simulink model "AeroPistonEngineSimulator"  (R2026a)
settings: Solver=VariableStepAuto  StopTime=100.0
model workspace (MAT data in the model file):
  linear_friction_constant = 0.001
undefined symbols (not defined in the file or in its folder): C_oil, CHT_capacity, EGT_tau, Fault_ID, friction_a, friction_b, J_engine, k_c, k_h, k_oil_cool, k_oil_heat, k_oil_pressure_rpm, k_oil_pressure_temp, RPM_max, T_max
libraries: simulink x17
settings Model: Creator=ambar  LastModifiedBy=skm
settings DataIOCC: LoadExternalInput=on

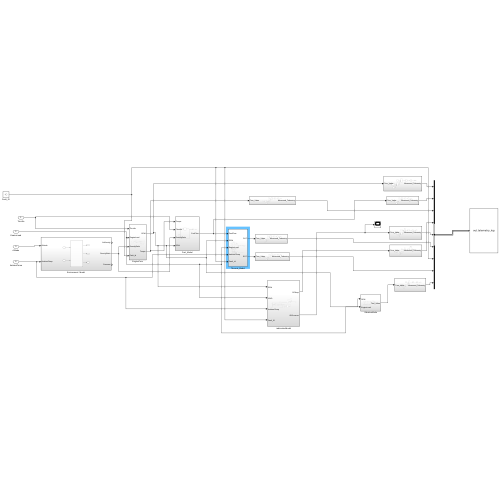
[thumbnail: Simulink's stored preview of the top-level diagram]
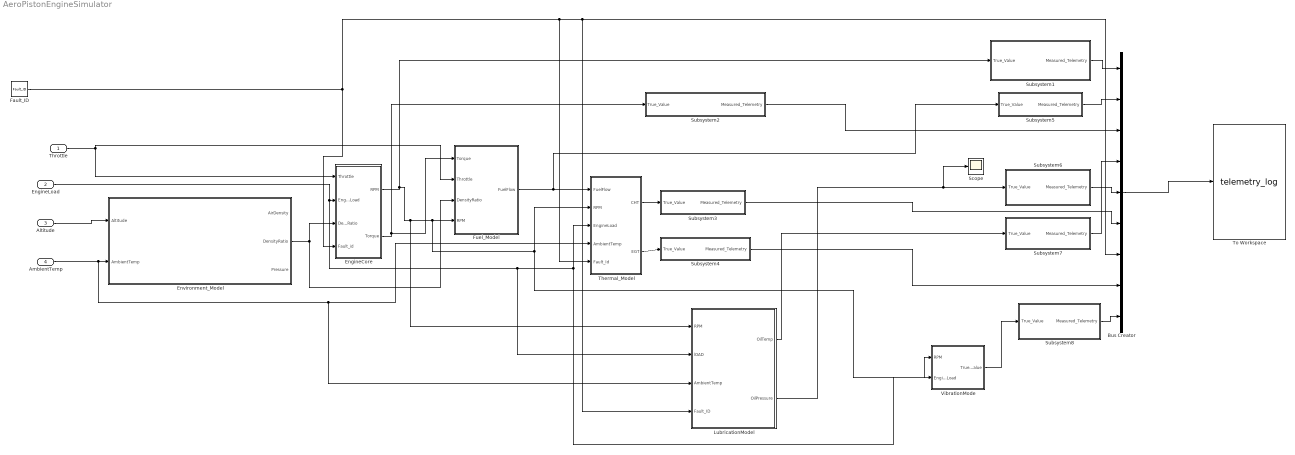
== system AeroPistonEngineSimulator ==
  Throttle : Inport
  EngineLoad : Inport  Port=2
  Altitude : Inport  Port=3
  AmbientTemp : Inport  Port=4
  Bus Creator : BusCreator  Inputs=9
  EngineCore : Subsystem
  Environment_Model : Subsystem
  Fault_ID : Constant  Value=Fault_ID
  Fuel_Model : Subsystem
  LubricationModel : Subsystem
  Scope : Scope
      settings: ActiveDisplayYMinimum=-7.3974032772630345  ActiveDisplayYMaximum=74.925308630368761  DataLoggingVariableName=ScopeData4
  Subsystem1 : Subsystem
  Subsystem2 : Subsystem
  Subsystem3 : Subsystem
  Subsystem4 : Subsystem
  Subsystem5 : Subsystem
  Subsystem6 : Subsystem
  Subsystem7 : Subsystem
  Subsystem8 : Subsystem
  Thermal_Model : Subsystem
  To Workspace : ToWorkspace  VariableName=telemetry_log  SaveFormat=Timeseries  SampleTime=-1
  VibrationMode : Subsystem
  wires:
  Altitude/1 -> Environment_Model/1(Altitude)
  AmbientTemp/1 -> LubricationModel/3(AmbientTemp), Thermal_Model/4(AmbientTemp), Environment_Model/2(AmbientTemp)
  Environment_Model/2(DensityRatio) -> Fuel_Model/3(DensityRatio), EngineCore/3(DensityRatio)
  EngineCore/1(RPM) -> Subsystem1/1(True_Value), LubricationModel/1(RPM), VibrationMode/1(RPM), Thermal_Model/2(RPM), Fuel_Model/4(RPM)
  EngineCore/2(Torque) -> Subsystem2/1(True_Value), Fuel_Model/1(Torque)
  Fuel_Model/1(FuelFlow) -> Subsystem5/1(True_Value), Thermal_Model/1(FuelFlow)
  Throttle/1 -> Fuel_Model/2(Throttle), EngineCore/1(Throttle)
  EngineLoad/1 -> LubricationModel/2(lOAD), Thermal_Model/3(EngineLoad), VibrationMode/2(EngineLoad), EngineCore/2(EngineLoad)
  Thermal_Model/1(CHT) -> Subsystem3/1(True_Value)
  Thermal_Model/2(EGT) -> Subsystem4/1(True_Value)
  LubricationModel/1(OilTemp) -> Subsystem7/1(True_Value)
  VibrationMode/1(True_Value) -> Subsystem8/1(True_Value)
  Subsystem8/1(Measured_Telemetry) -> Bus Creator/9
  Subsystem6/1(Measured_Telemetry) -> Bus Creator/5
  Subsystem7/1(Measured_Telemetry) -> Bus Creator/4
  Subsystem5/1(Measured_Telemetry) -> Bus Creator/2
  Subsystem1/1(Measured_Telemetry) -> Bus Creator/1
  Subsystem4/1(Measured_Telemetry) -> Bus Creator/8
  Subsystem3/1(Measured_Telemetry) -> Bus Creator/6
  Bus Creator/1 -> To Workspace/1
  Subsystem2/1(Measured_Telemetry) -> Bus Creator/3
  Fault_ID/1 -> Thermal_Model/5(Fault_Id), Bus Creator/7, LubricationModel/4(Fault_ID), EngineCore/4(Fault_id)
  LubricationModel/2(OilPressure) -> Scope/1, Subsystem6/1(True_Value)

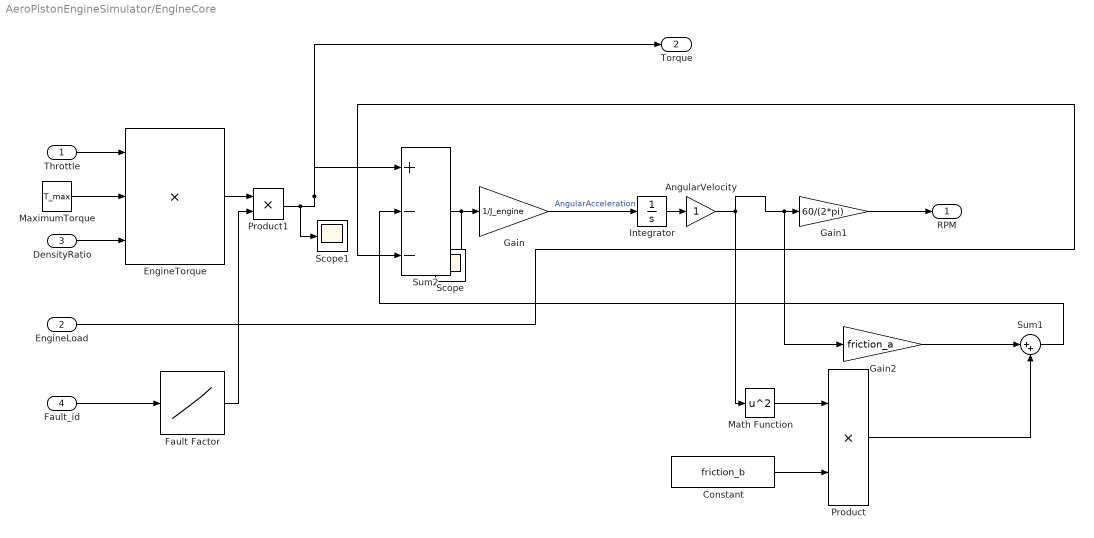
== system AeroPistonEngineSimulator/EngineCore ==
  Throttle : Inport
  EngineLoad : Inport  Port=2
  DensityRatio : Inport  Port=3
  Fault_id : Inport  Port=4
  AngularVelocity : Gain
  Constant : Constant  Value=friction_b
  EngineTorque : Product  Inputs=3
  Fault Factor : Lookup_n-D  NumberOfTableDimensions=1  BreakpointsForDimension1=[0 1 2 3 4]  Table=[1 0.65 1 1 1]  InternalRulePriority=Speed  RndMeth=Simplest
  Gain : Gain  Gain=1/J_engine
  Gain1 : Gain  Gain=60/(2*pi)
  Gain2 : Gain  Gain=friction_a
  Integrator : Integrator
  Math Function : Math  Operator=square
  MaximumTorque : Constant  Value=T_max  VectorParams1D=off
  Product : Product
  Product1 : Product
  Scope : Scope
      settings: ActiveDisplayYMinimum=-1.14558689108388  ActiveDisplayYMaximum=10.310282019757746  DataLoggingVariableName=ScopeData5
  Scope1 : Scope
      settings: ActiveDisplayYMinimum=-1  ActiveDisplayYMaximum=1  DataLoggingVariableName=ScopeData6
  Sum1 : Sum  Inputs=|++
  Sum2 : Sum  Inputs=|+--
  RPM : Outport
  Torque : Outport  Port=2
  wires:
  Throttle/1 -> EngineTorque/1
  DensityRatio/1 -> EngineTorque/3
  MaximumTorque/1 -> EngineTorque/2
  EngineTorque/1 -> Product1/1
  EngineLoad/1 -> Sum2/3
  Sum2/1 -> Scope/1, Gain/1
  Gain/1 -> Integrator/1  "AngularAcceleration"
  Gain1/1 -> RPM/1
  Integrator/1 -> AngularVelocity/1
  AngularVelocity/1 -> Gain1/1, Gain2/1, Math Function/1
  Math Function/1 -> Product/1
  Constant/1 -> Product/2
  Gain2/1 -> Sum1/1
  Product/1 -> Sum1/2
  Sum1/1 -> Sum2/2
  Fault_id/1 -> Fault Factor/1
  Product1/1 -> Scope1/1, Torque/1, Sum2/1
  Fault Factor/1 -> Product1/2

== system AeroPistonEngineSimulator/Environment_Model ==
  Altitude : Inport
  AmbientTemp : Inport  Port=2
  MATLAB Function : MATLAB Function  TreatAsAtomicUnit=on
  AirDensity : Outport
  DensityRatio : Outport  Port=2
  Pressure : Outport  Port=3
  wires:
  Altitude/1 -> MATLAB Function/1(altitude)
  AmbientTemp/1 -> MATLAB Function/2(temp_celsius)
  MATLAB Function/2(density) -> AirDensity/1
  MATLAB Function/3(density_ratio) -> DensityRatio/1
  MATLAB Function/1(pressure) -> Pressure/1

== system AeroPistonEngineSimulator/Fuel_Model ==
  Torque : Inport
  Throttle : Inport  Port=2
  DensityRatio : Inport  Port=3
  RPM : Inport  Port=4
  2-D Lookup Table : Lookup_n-D  BreakpointsForDimension1=[1500, 3000, 5000, 7000]  BreakpointsForDimension2=[0.2, 0.5, 0.8, 1.0]  Table=[0.5 0.8 1.2 1.5; 1.0 1.5 2.0 2.5; 1.8 2.2 2.8 3.5; 2.5 3.0 3.8 4.5]  InternalRulePriority=Speed  RndMeth=Simplest
      settings: InputPortMap=u0,u1
  Product : Product
  FuelFlow : Outport
  wires:
  RPM/1 -> 2-D Lookup Table/1
  Throttle/1 -> 2-D Lookup Table/2
  2-D Lookup Table/1 -> Product/1
  DensityRatio/1 -> Product/2
  Product/1 -> FuelFlow/1

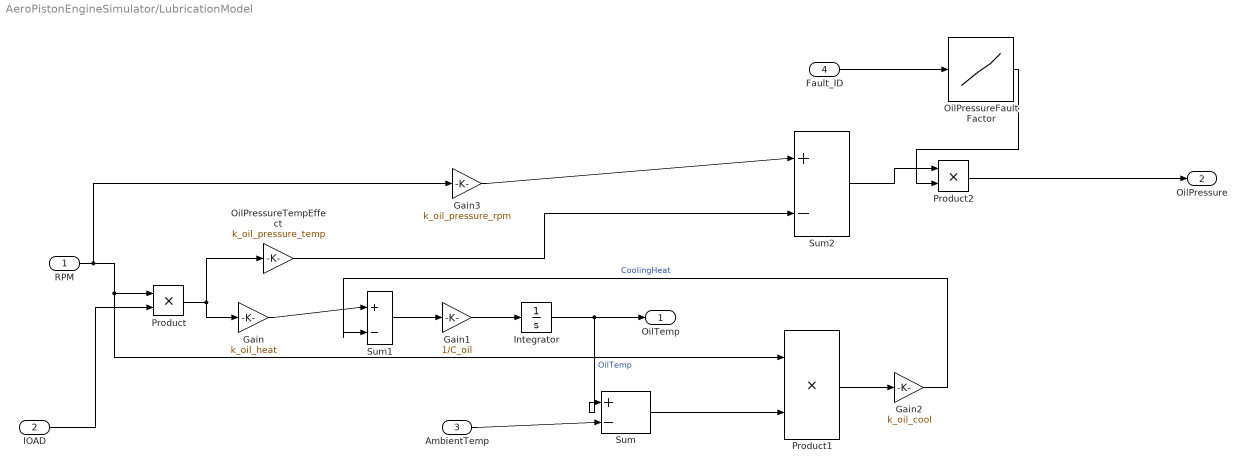
== system AeroPistonEngineSimulator/LubricationModel ==
  RPM : Inport
  lOAD : Inport  Port=2
  AmbientTemp : Inport  Port=3
  Fault_ID : Inport  Port=4
  Gain : Gain  Gain=k_oil_heat
  Gain1 : Gain  Gain=1/C_oil
  Gain2 : Gain  Gain=k_oil_cool
  Gain3 : Gain  Gain=k_oil_pressure_rpm
  Integrator : Integrator  InitialCondition=25
  OilPressureFault Factor : Lookup_n-D  NumberOfTableDimensions=1  BreakpointsForDimension1=[0 1 2 3 4]  Table=[1 1 1 0.2 1]  InternalRulePriority=Speed  RndMeth=Simplest
  OilPressureTempEffect : Gain  Gain=k_oil_pressure_temp
  Product : Product
  Product1 : Product
  Product2 : Product
  Sum : Sum  Inputs=|+-
  Sum1 : Sum  Inputs=|+-
  Sum2 : Sum  Inputs=|+-
  OilTemp : Outport
  OilPressure : Outport  Port=2
  wires:
  RPM/1 -> Gain3/1, Product1/1, Product/1
  lOAD/1 -> Product/2
  Product/1 -> OilPressureTempEffect/1, Gain/1
  AmbientTemp/1 -> Sum/2
  Gain/1 -> Sum1/1
  Sum1/1 -> Gain1/1
  Gain1/1 -> Integrator/1
  Integrator/1 -> Sum/1, OilTemp/1  "OilTemp"
  Sum/1 -> Product1/2
  Product1/1 -> Gain2/1
  Gain2/1 -> Sum1/2  "CoolingHeat"
  Gain3/1 -> Sum2/1
  Product2/1 -> OilPressure/1
  OilPressureTempEffect/1 -> Sum2/2
  Sum2/1 -> Product2/1
  Fault_ID/1 -> OilPressureFault Factor/1
  OilPressureFault Factor/1 -> Product2/2

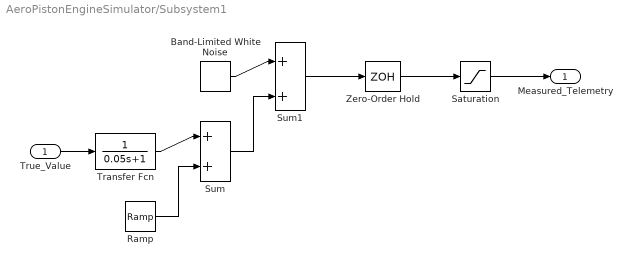
== system AeroPistonEngineSimulator/Subsystem1 ==
  True_Value : Inport
  Band-Limited White Noise : simulink/Sources/Band-Limited White Noise  Cov=[0.01]  Ts=0.1  seed=[23341]
  Ramp : simulink/Sources/Ramp  slope=0  start=0  InitialOutput=0
  Saturation : Saturate  UpperLimit=9000  LowerLimit=0
  Sum : Sum  Inputs=|++
  Sum1 : Sum  Inputs=|++
  Transfer Fcn : TransferFcn  Denominator=[0.05 1]
  Zero-Order Hold : ZeroOrderHold  SampleTime=0.05
  Measured_Telemetry : Outport
  wires:
  True_Value/1 -> Transfer Fcn/1
  Transfer Fcn/1 -> Sum/1
  Ramp/1 -> Sum/2
  Band-Limited White Noise/1 -> Sum1/1
  Sum/1 -> Sum1/2
  Sum1/1 -> Zero-Order Hold/1
  Zero-Order Hold/1 -> Saturation/1
  Saturation/1 -> Measured_Telemetry/1

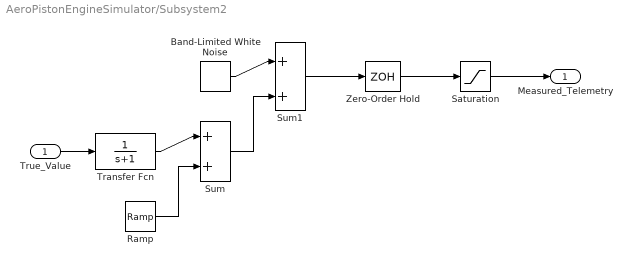
== system AeroPistonEngineSimulator/Subsystem2 ==
  True_Value : Inport
  Band-Limited White Noise : simulink/Sources/Band-Limited White Noise  Cov=[0.1]  Ts=0.1  seed=[23341]
  Ramp : simulink/Sources/Ramp  slope=0.001  start=0  InitialOutput=0
  Saturation : Saturate  UpperLimit=10  LowerLimit=-10
  Sum : Sum  Inputs=|++
  Sum1 : Sum  Inputs=|++
  Transfer Fcn : TransferFcn  Denominator=[1 1]
  Zero-Order Hold : ZeroOrderHold  SampleTime=-1
  Measured_Telemetry : Outport
  wires:
  True_Value/1 -> Transfer Fcn/1
  Transfer Fcn/1 -> Sum/1
  Ramp/1 -> Sum/2
  Band-Limited White Noise/1 -> Sum1/1
  Sum/1 -> Sum1/2
  Sum1/1 -> Zero-Order Hold/1
  Zero-Order Hold/1 -> Saturation/1
  Saturation/1 -> Measured_Telemetry/1

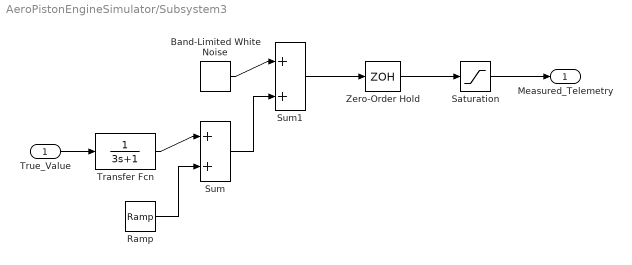
== system AeroPistonEngineSimulator/Subsystem3 ==
  True_Value : Inport
  Band-Limited White Noise : simulink/Sources/Band-Limited White Noise  Cov=0.05  Ts=0.1  seed=[23341]
  Ramp : simulink/Sources/Ramp  slope=0.001  start=0  InitialOutput=0
  Saturation : Saturate  UpperLimit=300  LowerLimit=0
  Sum : Sum  Inputs=|++
  Sum1 : Sum  Inputs=|++
  Transfer Fcn : TransferFcn  Denominator=[3 1]
  Zero-Order Hold : ZeroOrderHold  SampleTime=0.5
  Measured_Telemetry : Outport
  wires:
  True_Value/1 -> Transfer Fcn/1
  Transfer Fcn/1 -> Sum/1
  Ramp/1 -> Sum/2
  Band-Limited White Noise/1 -> Sum1/1
  Sum/1 -> Sum1/2
  Sum1/1 -> Zero-Order Hold/1
  Zero-Order Hold/1 -> Saturation/1
  Saturation/1 -> Measured_Telemetry/1

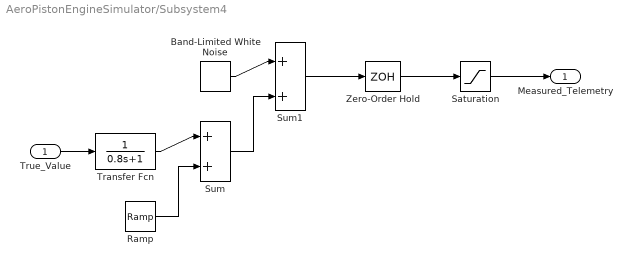
== system AeroPistonEngineSimulator/Subsystem4 ==
  True_Value : Inport
  Band-Limited White Noise : simulink/Sources/Band-Limited White Noise  Cov=[0.2]  Ts=0.1  seed=[23341]
  Ramp : simulink/Sources/Ramp  slope=1  start=0  InitialOutput=0
  Saturation : Saturate  UpperLimit=1000  LowerLimit=0
  Sum : Sum  Inputs=|++
  Sum1 : Sum  Inputs=|++
  Transfer Fcn : TransferFcn  Denominator=[0.8 1]
  Zero-Order Hold : ZeroOrderHold  SampleTime=0.1
  Measured_Telemetry : Outport
  wires:
  True_Value/1 -> Transfer Fcn/1
  Transfer Fcn/1 -> Sum/1
  Ramp/1 -> Sum/2
  Band-Limited White Noise/1 -> Sum1/1
  Sum/1 -> Sum1/2
  Sum1/1 -> Zero-Order Hold/1
  Zero-Order Hold/1 -> Saturation/1
  Saturation/1 -> Measured_Telemetry/1

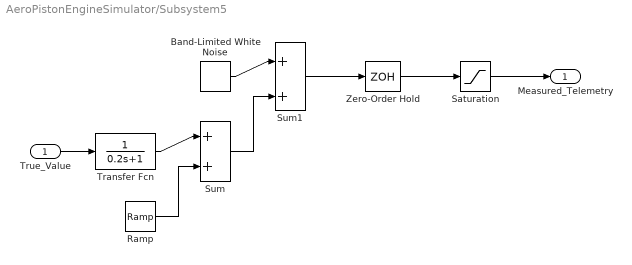
== system AeroPistonEngineSimulator/Subsystem5 ==
  True_Value : Inport
  Band-Limited White Noise : simulink/Sources/Band-Limited White Noise  Cov=[0.001]  Ts=0.1  seed=[23341]
  Ramp : simulink/Sources/Ramp  slope=0  start=0  InitialOutput=0
  Saturation : Saturate  UpperLimit=10  LowerLimit=0
  Sum : Sum  Inputs=|++
  Sum1 : Sum  Inputs=|++
  Transfer Fcn : TransferFcn  Denominator=[0.2 1]
  Zero-Order Hold : ZeroOrderHold  SampleTime=0.2
  Measured_Telemetry : Outport
  wires:
  True_Value/1 -> Transfer Fcn/1
  Transfer Fcn/1 -> Sum/1
  Ramp/1 -> Sum/2
  Band-Limited White Noise/1 -> Sum1/1
  Sum/1 -> Sum1/2
  Sum1/1 -> Zero-Order Hold/1
  Zero-Order Hold/1 -> Saturation/1
  Saturation/1 -> Measured_Telemetry/1

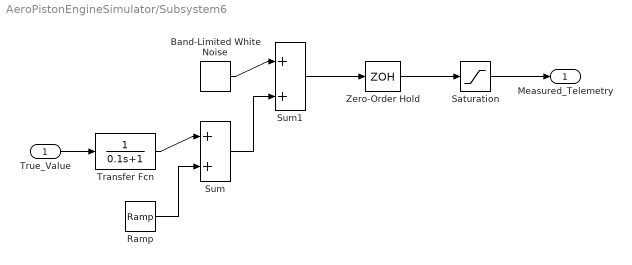
== system AeroPistonEngineSimulator/Subsystem6 ==
  True_Value : Inport
  Band-Limited White Noise : simulink/Sources/Band-Limited White Noise  Cov=0.05  Ts=0.1  seed=[23341]
  Ramp : simulink/Sources/Ramp  slope=-0.0005  start=0  InitialOutput=0
  Saturation : Saturate  UpperLimit=150  LowerLimit=0
  Sum : Sum  Inputs=|++
  Sum1 : Sum  Inputs=|++
  Transfer Fcn : TransferFcn  Denominator=[0.1 1]
  Zero-Order Hold : ZeroOrderHold  SampleTime=0.1
  Measured_Telemetry : Outport
  wires:
  True_Value/1 -> Transfer Fcn/1
  Transfer Fcn/1 -> Sum/1
  Ramp/1 -> Sum/2
  Band-Limited White Noise/1 -> Sum1/1
  Sum/1 -> Sum1/2
  Sum1/1 -> Zero-Order Hold/1
  Zero-Order Hold/1 -> Saturation/1
  Saturation/1 -> Measured_Telemetry/1

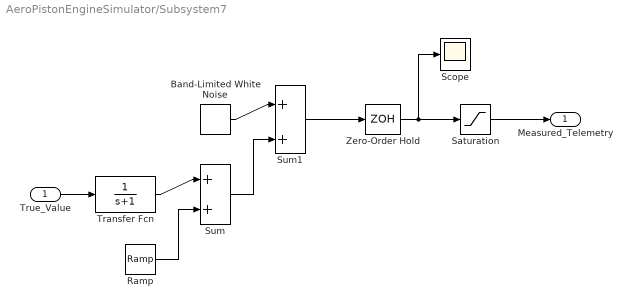
== system AeroPistonEngineSimulator/Subsystem7 ==
  True_Value : Inport
  Band-Limited White Noise : simulink/Sources/Band-Limited White Noise  Cov=[0.1]  Ts=0.1  seed=[23341]
  Ramp : simulink/Sources/Ramp  slope=0.001  start=0  InitialOutput=0
  Saturation : Saturate  UpperLimit=150  LowerLimit=0
  Scope : Scope
      settings: ActiveDisplayYMinimum=-75.19425986782052  ActiveDisplayYMaximum=450.06365181654218  DataLoggingVariableName=ScopeData3
  Sum : Sum  Inputs=|++
  Sum1 : Sum  Inputs=|++
  Transfer Fcn : TransferFcn  Denominator=[1 1]
  Zero-Order Hold : ZeroOrderHold  SampleTime=-1
  Measured_Telemetry : Outport
  wires:
  True_Value/1 -> Transfer Fcn/1
  Transfer Fcn/1 -> Sum/1
  Ramp/1 -> Sum/2
  Band-Limited White Noise/1 -> Sum1/1
  Sum/1 -> Sum1/2
  Sum1/1 -> Zero-Order Hold/1
  Zero-Order Hold/1 -> Scope/1, Saturation/1
  Saturation/1 -> Measured_Telemetry/1

== system AeroPistonEngineSimulator/Subsystem8 ==
  True_Value : Inport
  Band-Limited White Noise : simulink/Sources/Band-Limited White Noise  Cov=[0.1]  Ts=0.1  seed=[23341]
  Ramp : simulink/Sources/Ramp  slope=0  start=0  InitialOutput=0
  Saturation : Saturate  UpperLimit=20  LowerLimit=-20
  Sum : Sum  Inputs=|++
  Sum1 : Sum  Inputs=|++
  Transfer Fcn : TransferFcn  Denominator=[0.005 1]
  Zero-Order Hold : ZeroOrderHold  SampleTime=0.005
  Measured_Telemetry : Outport
  wires:
  True_Value/1 -> Transfer Fcn/1
  Transfer Fcn/1 -> Sum/1
  Ramp/1 -> Sum/2
  Band-Limited White Noise/1 -> Sum1/1
  Sum/1 -> Sum1/2
  Sum1/1 -> Zero-Order Hold/1
  Zero-Order Hold/1 -> Saturation/1
  Saturation/1 -> Measured_Telemetry/1

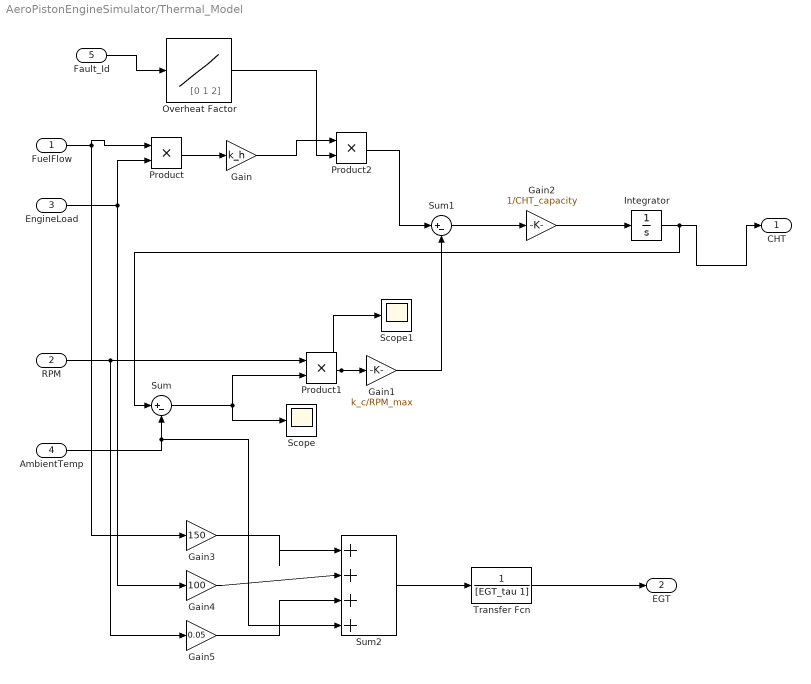
== system AeroPistonEngineSimulator/Thermal_Model ==
  note: [0 1 2]
  FuelFlow : Inport
  RPM : Inport  Port=2
  EngineLoad : Inport  Port=3
  AmbientTemp : Inport  Port=4
  Fault_Id : Inport  Port=5
  Gain : Gain  Gain=k_h
  Gain1 : Gain  Gain=k_c/RPM_max
  Gain2 : Gain  Gain=1/CHT_capacity
  Gain3 : Gain  Gain=150
  Gain4 : Gain  Gain=100
  Gain5 : Gain  Gain=0.05
  Integrator : Integrator  InitialCondition=25
  Overheat Factor : Lookup_n-D  NumberOfTableDimensions=1  BreakpointsForDimension1=[0 1 2 3 4]  Table=[1 1 2 1 1]  InternalRulePriority=Speed  RndMeth=Simplest
  Product : Product
  Product1 : Product
  Product2 : Product
  Scope : Scope
      settings: ActiveDisplayYMinimum=-1  ActiveDisplayYMaximum=1
  Scope1 : Scope
      settings: ActiveDisplayYMinimum=-9051.575897835155  ActiveDisplayYMaximum=81464.1830805164
  Sum : Sum  Inputs=|+-
  Sum1 : Sum  Inputs=|+-
  Sum2 : Sum  Inputs=|++++
  Transfer Fcn : TransferFcn  Denominator=[EGT_tau 1]
  CHT : Outport
  EGT : Outport  Port=2
  wires:
  FuelFlow/1 -> Product/1, Gain3/1
  EngineLoad/1 -> Gain4/1, Product/2
  Product/1 -> Gain/1
  AmbientTemp/1 -> Sum2/4, Sum/2
  RPM/1 -> Gain5/1, Product1/1
  Sum/1 -> Scope/1, Product1/2
  Product1/1 -> Scope1/1, Gain1/1
  Gain1/1 -> Sum1/2
  Gain/1 -> Product2/1
  Sum1/1 -> Gain2/1
  Integrator/1 -> CHT/1, Sum/1
  Gain2/1 -> Integrator/1
  Gain3/1 -> Sum2/1
  Gain4/1 -> Sum2/2
  Gain5/1 -> Sum2/3
  Sum2/1 -> Transfer Fcn/1
  Transfer Fcn/1 -> EGT/1
  Overheat Factor/1 -> Product2/2
  Fault_Id/1 -> Overheat Factor/1
  Product2/1 -> Sum1/1

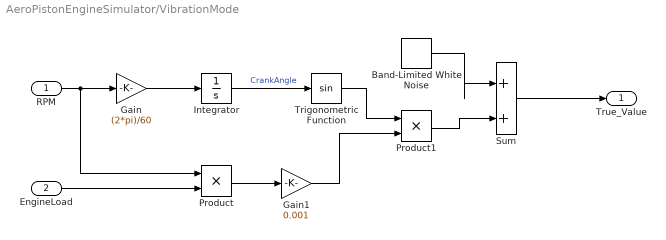
== system AeroPistonEngineSimulator/VibrationMode ==
  RPM : Inport
  EngineLoad : Inport  Port=2
  Band-Limited White Noise : simulink/Sources/Band-Limited White Noise  Cov=[0.1]  Ts=0.1  seed=[23341]
  Gain : Gain  Gain=(2*pi)/60
  Gain1 : Gain  Gain=0.001
  Integrator : Integrator
  Product : Product
  Product1 : Product
  Sum : Sum  Inputs=|++
  Trigonometric Function : Trigonometry
  True_Value : Outport
  wires:
  RPM/1 -> Product/1, Gain/1
  Gain/1 -> Integrator/1
  Integrator/1 -> Trigonometric Function/1  "CrankAngle"
  EngineLoad/1 -> Product/2
  Product/1 -> Gain1/1
  Trigonometric Function/1 -> Product1/1
  Gain1/1 -> Product1/2
  Product1/1 -> Sum/2
  Band-Limited White Noise/1 -> Sum/1
  Sum/1 -> True_Value/1

== matlab function AeroPistonEngineSimulator/Environment_Model/MATLAB Function ==
  data: altitude input; pressure output; temp_celsius input; density output; density_ratio output
function [pressure, density, density_ratio] = calculate_atmosphere(altitude, temp_celsius)
    % Standard ISA Constants
    P0 = 101325;       % Sea level standard pressure (Pa)
    T0 = 288.15;       % Sea level standard temperature (K)
    rho0 = 1.225;      % Sea level standard density (kg/m^3)
    L = 0.0065;        % Temperature lapse rate (K/m)
    R = 287.05;        % Specific gas constant for dry air (J/(kg*K))
    g = 9.80665;       % Gravity (m/s^2)
    
    % Convert input temp to Kelvin
    T_ambient = temp_celsius + 273.15;
    
    % Calculate pressure at altitude
    % Assuming troposphere (under ~11,000m)
    pressure = P0 * (1 - (L * altitude) / T0) ^ ((g) / (R * L));
    
    % Calculate current air density (Ideal Gas Law: P = rho * R * T)
    density = pressure / (R * T_ambient);
    
    % Calculate density ratio (sigma)
    density_ratio = density / rho0;
end
